simulink model "exp02"  (R2018a)
settings: Solver=VariableStepAuto  StartTime=0.0  StopTime=10.0  RelTol=1e-3
settings Model: Creator=Administrator  LastModifiedBy=Administrator

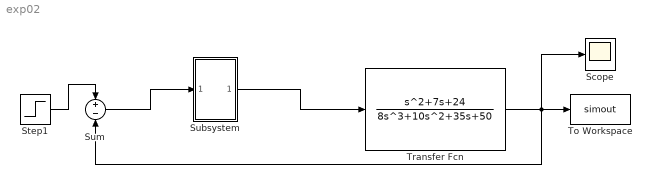
== system exp02 ==
  Scope : Scope
  Step1 : Step  SampleTime=0
  Subsystem : Subsystem
  Sum : Sum  Inputs=+-
  To Workspace : ToWorkspace  VariableName=simout  SampleTime=-1
  Transfer Fcn : TransferFcn  Numerator=[1 7 24]  Denominator=[8 10 35 50]
  wires:
  Transfer Fcn/1 -> Scope/1, To Workspace/1, Sum/2
  Step1/1 -> Sum/1
  Sum/1 -> Subsystem/1(In1)
  Subsystem/1(Out1) -> Transfer Fcn/1

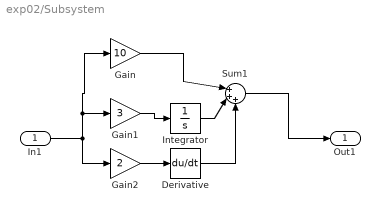
== system exp02/Subsystem ==
  In1 : Inport
  Derivative : Derivative
  Gain : Gain  Gain=10
      mask Display: disp('kp')
  Gain1 : Gain  Gain=3
      mask Display: disp('ki')
  Gain2 : Gain  Gain=2
      mask Display: disp('kd')
  Integrator : Integrator
  Sum1 : Sum  Inputs=|+++
  Out1 : Outport
  wires:
  Derivative/1 -> Sum1/3
  In1/1 -> Gain/1, Gain1/1, Gain2/1
  Gain1/1 -> Integrator/1
  Sum1/1 -> Out1/1
  Gain/1 -> Sum1/1
  Integrator/1 -> Sum1/2
  Gain2/1 -> Derivative/1
